simulink model "take2"  (R2021a)
settings: Solver=VariableStepAuto  StartTime=0.0  StopTime=3600  RelTol=1e-6
undefined symbols (not defined in the file): Ion, Lithium
libraries: spsVariableResistorLib x1, spsBatteryLib x1, spspowerguiLib x1
settings Model: Creator=sarah  LastModifiedBy=sarah

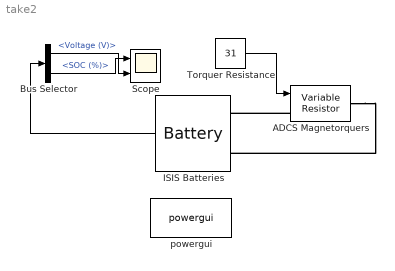
== system take2 ==
  ADCS Magnetorquers : spsVariableResistorLib/Variable Resistor  Rabsmin=31
      settings: SourceProductBaseCode=PS
  Bus Selector : BusSelector  OutputSignals=Voltage (V),SOC (%)
  ISIS Batteries : spsBatteryLib/Battery  BatType=Lithium-Ion  ShowTempParam=off  ThermalPreset=no  ShowAgeParam=off  NomV=16  NomQ=45/16  SOC=100  Batt_Tr=30  PresetModel=on  MaxQ=2.8125  MinV=12  FullV=18.6238  Dis_rate=1.2228  R=0.056889  Normal_OP=2.5435  expZone="[17.2862     0.138179]"  current=[6.5 13 32.5]  Units=Time  Tci=20  NomT=20  T2=-30  MaxQ2=4.8  FullV2=7.1  Normal_OP2=5.655  expZone2="[6.58           1]"  Rca=0.6  ti=2000  Dp=0  Neq0=0  Tsim=1e6  Ta1=25  Qeol=5.4*0.9  Reol=0.013333*1.2  Char_age=[2.3478, 3]  Dis_age=[2.3478, 10]  N1=1500  N2=10500  N3=1000  N4=1400  Ta2=45  N5=950
  Scope : Scope  NumInputPorts=2
  Torquer Resistance : Constant  Value=31
  powergui : spspowerguiLib/powergui  Priority=1  SimulationMode=Discrete  SampleTime=.05  frequency=60  Iterations=50  frequencyindice=0  Pbase=100e6  ErrMax=1e-4  UnitsV=kV  UnitsW=MW  buscounter=0  FunctionMessages=off  echomessages=off  EnableUseOfTLC=off  CurrentSourceSwitches=off  DisableSnubberDevices=off  DisableRonSwitches=off  DisableVfSwitches=off  DisplayEquations=off  AutomaticDiscreteSolvers=off  SolverType=Tustin/Backward Euler (TBE)  Interpol=off  ExternalGateDelay=off  methode=off  Ts=100  x0status=blocks  SPID=on  SwTol=0  HookPort=off  NonlinearTolerance=1e-4  nMaxIteration=100  ContinueOnMaxIteration=off  RestoreLinks=warning  ResistiveCurrentMeasurement=off  Frange=[0:2:500]  Ylog=off  Xlog=on  ShowGrid=off  save=off  variable=ZData  structure=0  ZoomFFT=off  StartTime=0.0  cycles=1  DisplayStyle=1  fundamental=60  FreqAxis=off  MaxFrequency=1000  frequencyindicesteady=1  RmsSteady=1  display=off
  wires:
  Torquer Resistance/1 -> ADCS Magnetorquers/1
  ISIS Batteries/1 -> Bus Selector/1
  Bus Selector/1 -> Scope/2  "<Voltage (V)>"
  Bus Selector/2 -> Scope/1  "<SOC (%)>"
  connections:
  ADCS Magnetorquers/LConn1 -- ISIS Batteries/LConn1
  ADCS Magnetorquers/RConn1 -- ISIS Batteries/LConn2
